simulink model "gm_sampleModel1954_3_sub"  (R2023a)
settings: Solver=VariableStepAuto  StartTime=0.0  StopTime=10.0  RelTol=1e-3
libraries: simulink x1
settings Model: Creator=user1  LastModifiedBy=user1
settings OptimizationCC: BlockReduction=off  ConditionallyExecuteInputs=off
settings DebuggingCC: InheritedTsInSrcMsg=none

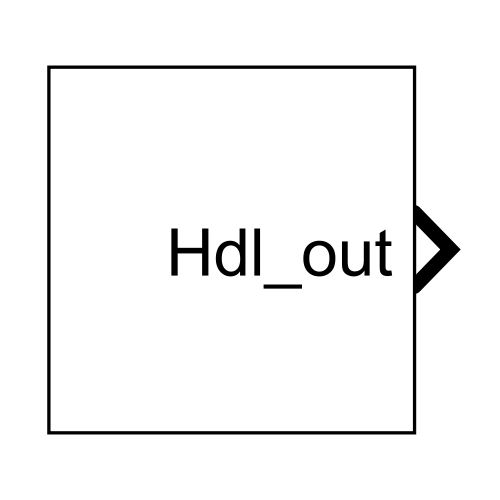
[thumbnail: Simulink's stored preview of the top-level diagram]
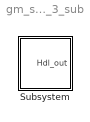
== system gm_sampleModel1954_3_sub ==
  Subsystem : Subsystem

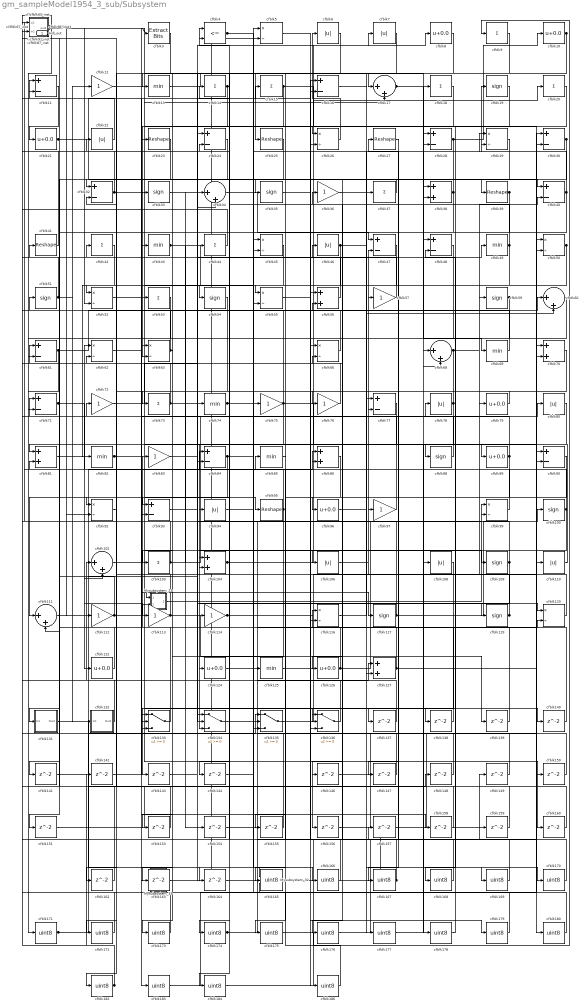
== system gm_sampleModel1954_3_sub/Subsystem ==
  Mysubsystem_23 : Subsystem
  Mysubsystem_32 : Subsystem
  Mysubsystem_33 : Subsystem
  cfblk{8,10,21,79,89,96,122,124,126} (9 alike) : Bias  Bias=0.0  SaturateOnIntegerOverflow=off
  cfblk{19,33,35,51,54,59,88,100,109,117,119} (11 alike) : Signum
  cfblk101_inst : Subsystem
  cfblk{17,34,60,68,102,111} (6 alike) : Sum  Inputs=|++  OutDataTypeStr=uint8
  cfblk{9,14..15,18,20,37,42,44,53,73,103} (11 alike) : Sum  Inputs=+  OutDataTypeStr=uint8
  cfblk{38,56,70,81,86,104,127} (7 alike) : Sum  OutDataTypeStr=uint8
  cfblk105_inst : Subsystem
  cfblk{6..7,22,46,78,80,94,106,108,110} (10 alike) : Abs  OutDataTypeStr=uint8  SaturateOnIntegerOverflow=off
  cfblk107_inst : Subsystem
  cfblk{11,16,24,28,30,32,40,47..48,61,71,77,84,90,93} (15 alike) : Sum  Inputs=+-  OutDataTypeStr=uint8
  cfblk{12,36,57,72,75..76,83,97,112..114} (11 alike) : Gain  OutDataTypeStr=uint8
  cfblk115_inst : Subsystem
  cfblk{5,26,29,45,50,52,55,62..63,66,92,99,116,120} (14 alike) : Product  Inputs=*/  OutDataTypeStr=uint8  RndMeth=Zero  SaturateOnIntegerOverflow=on
  cfblk118_inst : Subsystem
  cfblk121_inst : Subsystem
  cfblk{13,43,49,69,74,82,85,125} (8 alike) : MinMax  OutDataTypeStr=uint8
  cfblk129_inst : Subsystem
  cfblk131 : Subsystem
  cfblk132 : Subsystem
  cfblk{133..136} (4 alike) : Switch  OutDataTypeStr=uint8  SaturateOnIntegerOverflow=off  InputSameDT=off
  cfblk{137..144,146..151,153..160,162..164} (25 alike) : Delay  SampleTime=1
  cfblk{165..180,182..184,186} (20 alike) : DataTypeConversion  OutDataTypeStr=uint8  SaturateOnIntegerOverflow=off  RndMeth=Floor
  cfblk2 : Constant  Value=0  OutDataTypeStr=uint8  SampleTime=1
  cfblk{23,25,27,39,41,95} (6 alike) : Reshape
  cfblk3 : simulink/Logic and Bit Operations/Extract Bits  bitsToExtract=Upper half  numBits=8  bitIdxRange=[0 7]  outScalingMode=Preserve fixed-point scaling
      settings: LibrarySourceBlock=|
      | hdlsllib/Logic and Bit
      | Operations/Extract Bits
  cfblk31_inst : Subsystem
  cfblk4 : RelationalOperator  Operator=<=  OutDataTypeStr=boolean  InputSameDT=off
  cfblk58_inst : Subsystem
  cfblk64_inst : Subsystem
  cfblk65_inst : Subsystem
  cfblk67_inst : Subsystem
  cfblk87_inst : Subsystem
  cfblk91_inst : Subsystem
  cfblk98_inst : Subsystem
  Hdl_out : Outport  OutDataTypeStr=uint8  SampleTime=1
  wires:
  Mysubsystem_23/1(Out1) -> cfblk99/1
  Mysubsystem_32/1(Out1) -> cfblk159/1
  Mysubsystem_33/1(Out1) -> cfblk5/2
  cfblk10/1 -> cfblk25/1, cfblk55/1
  cfblk100/1 -> cfblk134/3, cfblk129_inst/1(in1)
  cfblk101_inst/1(out1) -> cfblk118_inst/1(in1)
  cfblk102/1 -> cfblk140/1
  cfblk103/1 -> cfblk78/1, cfblk58_inst/2(in2), cfblk34/1
  cfblk104/1 -> cfblk7/1, cfblk20/1
  cfblk105_inst/1(out1) -> cfblk95/1, cfblk106/1, cfblk55/2
  cfblk106/1 -> cfblk47/2
  cfblk107_inst/1(out1) -> cfblk137/1
  cfblk108/1 -> cfblk143/1
  cfblk109/1 -> cfblk124/1, cfblk105_inst/2(in2)
  cfblk11/1 -> cfblk21/1
  cfblk110/1 -> cfblk89/1
  cfblk111/1 -> cfblk86/1
  cfblk112/1 -> cfblk11/1, cfblk138/1
  cfblk113/1 -> cfblk107_inst/2(in2), cfblk139/1
  cfblk114/1 -> cfblk79/1, cfblk68/1
  cfblk115_inst/1(out1) -> cfblk91_inst/2(in2), cfblk26/1
  cfblk116/1 -> cfblk37/1
  cfblk117/1 -> cfblk121_inst/2(in2), cfblk100/1
  cfblk118_inst/1(out1) -> cfblk17/2, cfblk156/1
  cfblk119/1 -> cfblk97/1, cfblk57/1
  cfblk12/1 -> cfblk160/1
  cfblk120/1 -> cfblk72/1
  cfblk121_inst/1(out1) -> cfblk109/1
  cfblk122/1 -> cfblk71/1
  cfblk124/1 -> cfblk120/2
  cfblk125/1 -> cfblk90/1
  cfblk126/1 -> cfblk68/2, cfblk64_inst/1(in1)
  cfblk127/1 -> cfblk30/1, cfblk83/1
  cfblk129_inst/1(out1) -> cfblk180/1, cfblk104/2
  cfblk13/1 -> cfblk17/1
  cfblk131/1(Out1) -> cfblk164/1
  cfblk132/1(Out1) -> cfblk61/1
  cfblk133/1 -> cfblk107_inst/1(in1)
  cfblk134/1 -> cfblk18/1
  cfblk135/1 -> cfblk59/1
  cfblk136/1 -> cfblk102/1
  cfblk137/1 -> cfblk129_inst/2(in2)
  cfblk138/1 -> cfblk116/1
  cfblk139/1 -> cfblk81/2
  cfblk14/1 -> cfblk63/2, cfblk144/1
  cfblk140/1 -> cfblk11/2
  cfblk141/1 -> cfblk34/2
  cfblk142/1 -> cfblk77/2
  cfblk143/1 -> cfblk56/2
  cfblk144/1 -> cfblk45/2
  cfblk146/1 -> cfblk38/1
  cfblk147/1 -> cfblk62/2
  cfblk148/1 -> cfblk118_inst/2(in2)
  cfblk149/1 -> cfblk31_inst/2(in2)
  cfblk15/1 -> cfblk90/2, cfblk23/1
  cfblk150/1 -> cfblk86/2
  cfblk151/1 -> cfblk134/1
  cfblk153/1 -> cfblk32/2
  cfblk154/1 -> cfblk127/1
  cfblk155/1 -> cfblk84/1
  cfblk156/1 -> cfblk50/2
  cfblk157/1 -> cfblk30/2
  cfblk158/1 -> cfblk111/2
  cfblk159/1 -> cfblk115_inst/2(in2)
  cfblk16/1 -> cfblk60/2
  cfblk160/1 -> cfblk66/2
  cfblk162/1 -> cfblk105_inst/1(in1)
  cfblk163/1 -> cfblk99/2
  cfblk164/1 -> cfblk26/2
  cfblk165/1 -> cfblk108/1
  cfblk166/1 -> cfblk85/1
  cfblk167/1 -> cfblk67_inst/2(in2), cfblk46/1, cfblk14/1
  cfblk168/1 -> cfblk27/1
  cfblk169/1 -> cfblk56/1
  cfblk17/1 -> cfblk28/1, cfblk69/1
  cfblk170/1 -> cfblk36/1
  cfblk171/1 -> cfblk135/1, cfblk148/1
  cfblk172/1 -> cfblk65_inst/1(in1)
  cfblk173/1 -> cfblk65_inst/2(in2)
  cfblk174/1 -> cfblk110/1, cfblk157/1
  cfblk175/1 -> cfblk9/1
  cfblk176/1 -> cfblk149/1
  cfblk177/1 -> cfblk48/1
  cfblk178/1 -> cfblk48/2
  cfblk179/1 -> cfblk115_inst/1(in1)
  cfblk18/1 -> cfblk127/2
  cfblk180/1 -> cfblk5/1
  cfblk182/1 -> cfblk101_inst/1(in1), cfblk142/1
  cfblk183/1 -> cfblk70/1
  cfblk184/1 -> cfblk70/2
  cfblk186/1 -> Mysubsystem_32/2(In2)
  cfblk19/1 -> cfblk168/1
  cfblk2/1 -> cfblk98_inst/2(in2), cfblk92/2, cfblk112/1
  cfblk20/1 -> cfblk153/1
  cfblk21/1 -> cfblk38/2, cfblk15/1
  cfblk22/1 -> cfblk67_inst/1(in1)
  cfblk23/1 -> cfblk53/1
  cfblk24/1 -> cfblk162/1
  cfblk25/1 -> cfblk141/1
  cfblk26/1 -> cfblk6/1
  cfblk27/1 -> cfblk167/1
  cfblk28/1 -> cfblk133/3, cfblk10/1
  cfblk29/1 -> cfblk39/1
  cfblk3/1 -> cfblk13/1
  cfblk30/1 -> cfblk96/1, cfblk81/1
  cfblk31_inst/1(out1) -> cfblk186/1, cfblk114/1
  cfblk32/1 -> cfblk98_inst/1(in1), cfblk54/1, cfblk172/1, cfblk75/1
  cfblk33/1 -> cfblk119/1
  cfblk34/1 -> cfblk77/1
  cfblk35/1 -> cfblk47/1
  cfblk36/1 -> cfblk169/1
  cfblk37/1 -> cfblk33/1
  cfblk38/1 -> cfblk35/1, cfblk134/2
  cfblk39/1 -> cfblk135/2, cfblk151/1
  cfblk4/1 -> cfblk40/1, cfblk166/1
  cfblk40/1 -> cfblk19/1, cfblk104/1
  cfblk41/1 -> cfblk31_inst/1(in1)
  cfblk42/1 -> cfblk82/1
  cfblk43/1 -> cfblk135/3, cfblk154/1, cfblk125/1
  cfblk44/1 -> cfblk87_inst/2(in2)
  cfblk45/1 -> cfblk94/1
  cfblk46/1 -> cfblk29/2, cfblk150/1, Mysubsystem_23/1(In1)
  cfblk47/1 -> cfblk93/1
  cfblk48/1 -> cfblk176/1
  cfblk49/1 -> cfblk22/1, cfblk52/1
  cfblk5/1 -> cfblk179/1
  cfblk50/1 -> cfblk175/1, cfblk92/1, cfblk63/1
  cfblk51/1 -> cfblk64_inst/2(in2), cfblk12/1, cfblk132/1(In1)
  cfblk52/1 -> cfblk183/1
  cfblk53/1 -> cfblk61/2
  cfblk54/1 -> cfblk103/1
  cfblk55/1 -> cfblk16/2
  cfblk56/1 -> cfblk41/1
  cfblk57/1 -> cfblk24/2
  cfblk58_inst/1(out1) -> Mysubsystem_33/1(In1)
  cfblk59/1 -> cfblk136/2, cfblk147/1, cfblk146/1
  cfblk6/1 -> cfblk32/1
  cfblk60/1 -> cfblk133/2
  cfblk61/1 -> cfblk71/2, cfblk50/1
  cfblk62/1 -> cfblk117/1
  cfblk63/1 -> cfblk58_inst/1(in1), cfblk173/1
  cfblk64_inst/1(out1) -> cfblk121_inst/1(in1), Mysubsystem_23/2(In2)
  cfblk65_inst/1(out1) -> cfblk171/1
  cfblk66/1 -> cfblk51/1
  cfblk67_inst/1(out1) -> cfblk74/1
  cfblk68/1 -> cfblk88/1, cfblk40/2, cfblk184/1
  cfblk69/1 -> cfblk4/1
  cfblk7/1 -> cfblk43/1
  cfblk70/1 -> cfblk182/1
  cfblk71/1 -> cfblk102/2, cfblk113/1
  cfblk72/1 -> cfblk44/1
  cfblk73/1 -> cfblk101_inst/2(in2), cfblk49/1
  cfblk74/1 -> cfblk136/1, cfblk120/1
  cfblk75/1 -> cfblk4/2, cfblk178/1, cfblk131/1(In1)
  cfblk76/1 -> cfblk87_inst/1(in1)
  cfblk77/1 -> cfblk84/2
  cfblk78/1 -> cfblk126/1, cfblk76/1
  cfblk79/1 -> cfblk73/1
  cfblk8/1 -> cfblk133/1
  cfblk80/1 -> cfblk93/2
  cfblk81/1 -> cfblk122/1
  cfblk82/1 -> cfblk16/1, cfblk158/1, Mysubsystem_32/1(In1)
  cfblk83/1 -> cfblk80/1
  cfblk84/1 -> cfblk111/1, cfblk29/1
  cfblk85/1 -> cfblk165/1
  cfblk86/1 -> cfblk116/2
  cfblk87_inst/1(out1) -> cfblk177/1
  cfblk88/1 -> cfblk66/1
  cfblk89/1 -> cfblk91_inst/1(in1), cfblk136/3
  cfblk9/1 -> cfblk174/1
  cfblk90/1 -> cfblk155/1
  cfblk91_inst/1(out1) -> cfblk28/2, cfblk52/2
  cfblk92/1 -> cfblk42/1
  cfblk93/1 -> cfblk8/1
  cfblk94/1 -> cfblk60/1
  cfblk95/1 -> cfblk24/1, cfblk163/1
  cfblk96/1 -> cfblk170/1
  cfblk97/1 -> cfblk45/1
  cfblk98_inst/1(out1) -> cfblk3/1, Hdl_out/1
  cfblk99/1 -> cfblk62/1

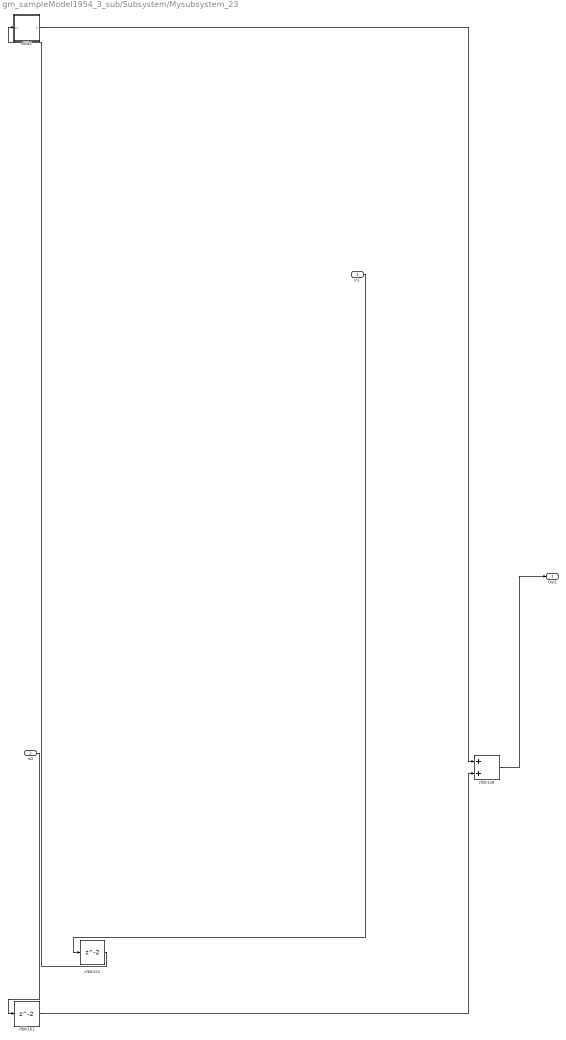
== system gm_sampleModel1954_3_sub/Subsystem/Mysubsystem_23 ==
  In1 : Inport  OutDataTypeStr=uint8  PortDimensions=1  SampleTime=1
  In2 : Inport  Port=2  OutDataTypeStr=uint8  PortDimensions=1  SampleTime=1
  cfblk1 : Subsystem  mask(Detect Fall Nonpositive){vinit=double(0), InputProcessing=Elements as channels (sample based), OutDataTypeStr=boolean}
      mask prompts: vinit "Simulink:masks:InitialCondition_MP"; InputProcessing "Simulink:masks:InputProcessing_MP"; OutDataTypeStr "Simulink:masks:OutputDataType_MP"
      mask help: Simulink:masks:DetectFallNonpositive_MD
      mask init:
      | InputProcessing = 'Elements as channels (sample based)';
      | OutDataTypeStr = 'boolean';
      | vinit = double(0);
      mask TypeOptions InputProcessing: Simulink:masks:ColumnsAsChannelsFrameBased | Simulink:masks:ElementsAsChannelsSampleBased
      mask TypeOptions OutDataTypeStr: Simulink:masks:uint8 | Simulink:masks:boolean
      mask Display: fprintf('U <= 0\n&  NOT\nU/z <= 0')
  cfblk128 : Sum
  cfblk152 : Delay  SampleTime=1
  cfblk161 : Delay  SampleTime=1
  Out1 : Outport  SampleTime=1
  wires:
  In1/1 -> cfblk152/1
  In2/1 -> cfblk161/1
  cfblk1/1(Y) -> cfblk128/1
  cfblk128/1 -> Out1/1
  cfblk152/1 -> cfblk1/1(U)
  cfblk161/1 -> cfblk128/2

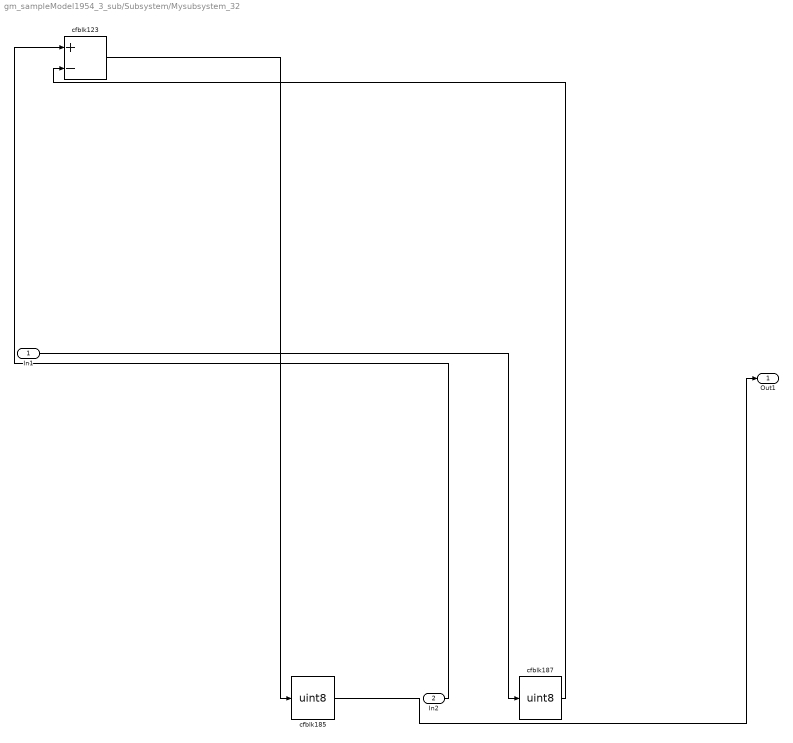
== system gm_sampleModel1954_3_sub/Subsystem/Mysubsystem_32 ==
  In1 : Inport  OutDataTypeStr=uint8  PortDimensions=1  SampleTime=1
  In2 : Inport  Port=2  OutDataTypeStr=uint8  PortDimensions=1  SampleTime=1
  cfblk123 : Sum  Inputs=+-
  cfblk185 : DataTypeConversion  OutDataTypeStr=uint8  SaturateOnIntegerOverflow=off  RndMeth=Floor
  cfblk187 : DataTypeConversion  OutDataTypeStr=uint8  SaturateOnIntegerOverflow=off  RndMeth=Floor
  Out1 : Outport  SampleTime=1
  wires:
  In1/1 -> cfblk187/1
  In2/1 -> cfblk123/1
  cfblk123/1 -> cfblk185/1
  cfblk185/1 -> Out1/1
  cfblk187/1 -> cfblk123/2

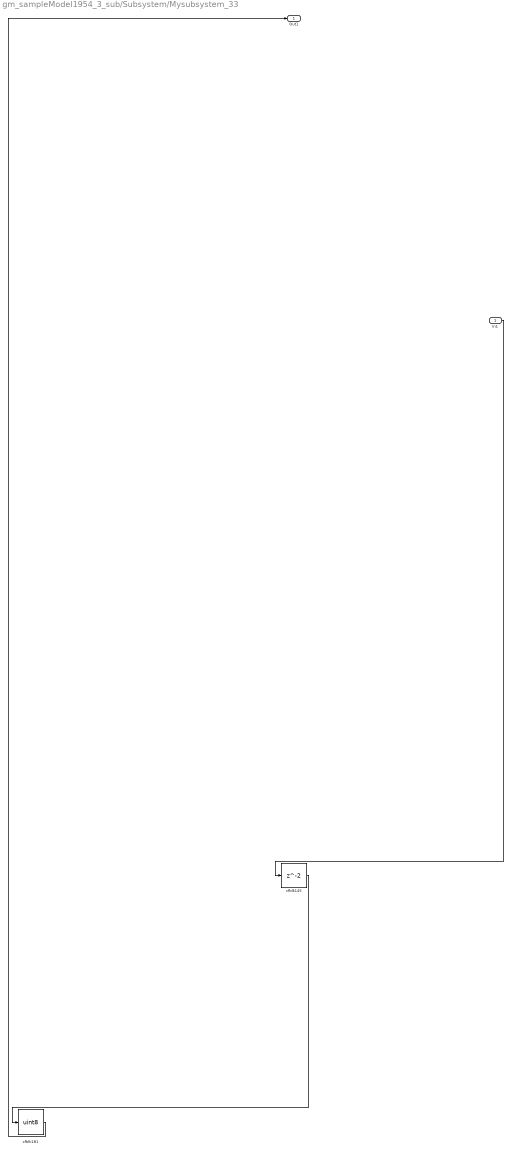
== system gm_sampleModel1954_3_sub/Subsystem/Mysubsystem_33 ==
  In1 : Inport  OutDataTypeStr=uint8  PortDimensions=1  SampleTime=1
  cfblk145 : Delay  SampleTime=1
  cfblk181 : DataTypeConversion  OutDataTypeStr=uint8  SaturateOnIntegerOverflow=off  RndMeth=Floor
  Out1 : Outport  SampleTime=1
  wires:
  In1/1 -> cfblk145/1
  cfblk145/1 -> cfblk181/1
  cfblk181/1 -> Out1/1

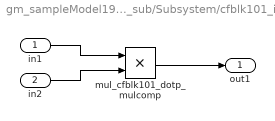
== system gm_sampleModel1954_3_sub/Subsystem/cfblk101_inst ==
  in1 : Inport  OutDataTypeStr=uint8  SampleTime=1
  in2 : Inport  Port=2  OutDataTypeStr=uint8  SampleTime=1
  mul_cfblk101_dotp_mulcomp : Product  Inputs=**  OutDataTypeStr=uint8  SampleTime=1
  out1 : Outport  OutDataTypeStr=uint8  SampleTime=1
  wires:
  in1/1 -> mul_cfblk101_dotp_mulcomp/1
  in2/1 -> mul_cfblk101_dotp_mulcomp/2
  mul_cfblk101_dotp_mulcomp/1 -> out1/1

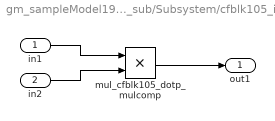
== system gm_sampleModel1954_3_sub/Subsystem/cfblk105_inst ==
  in1 : Inport  OutDataTypeStr=uint8  SampleTime=1
  in2 : Inport  Port=2  OutDataTypeStr=uint8  SampleTime=1
  mul_cfblk105_dotp_mulcomp : Product  Inputs=**  OutDataTypeStr=uint8  SampleTime=1
  out1 : Outport  OutDataTypeStr=uint8  SampleTime=1
  wires:
  in1/1 -> mul_cfblk105_dotp_mulcomp/1
  in2/1 -> mul_cfblk105_dotp_mulcomp/2
  mul_cfblk105_dotp_mulcomp/1 -> out1/1

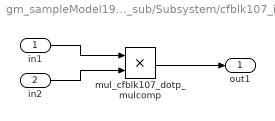
== system gm_sampleModel1954_3_sub/Subsystem/cfblk107_inst ==
  in1 : Inport  OutDataTypeStr=uint8  SampleTime=1
  in2 : Inport  Port=2  OutDataTypeStr=uint8  SampleTime=1
  mul_cfblk107_dotp_mulcomp : Product  Inputs=**  OutDataTypeStr=uint8  SampleTime=1
  out1 : Outport  OutDataTypeStr=uint8  SampleTime=1
  wires:
  in1/1 -> mul_cfblk107_dotp_mulcomp/1
  in2/1 -> mul_cfblk107_dotp_mulcomp/2
  mul_cfblk107_dotp_mulcomp/1 -> out1/1

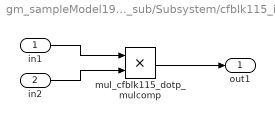
== system gm_sampleModel1954_3_sub/Subsystem/cfblk115_inst ==
  in1 : Inport  OutDataTypeStr=uint8  SampleTime=1
  in2 : Inport  Port=2  OutDataTypeStr=uint8  SampleTime=1
  mul_cfblk115_dotp_mulcomp : Product  Inputs=**  OutDataTypeStr=uint8  SampleTime=1
  out1 : Outport  OutDataTypeStr=uint8  SampleTime=1
  wires:
  in1/1 -> mul_cfblk115_dotp_mulcomp/1
  in2/1 -> mul_cfblk115_dotp_mulcomp/2
  mul_cfblk115_dotp_mulcomp/1 -> out1/1

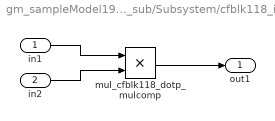
== system gm_sampleModel1954_3_sub/Subsystem/cfblk118_inst ==
  in1 : Inport  OutDataTypeStr=uint8  SampleTime=1
  in2 : Inport  Port=2  OutDataTypeStr=uint8  SampleTime=1
  mul_cfblk118_dotp_mulcomp : Product  Inputs=**  OutDataTypeStr=uint8  SampleTime=1
  out1 : Outport  OutDataTypeStr=uint8  SampleTime=1
  wires:
  in1/1 -> mul_cfblk118_dotp_mulcomp/1
  in2/1 -> mul_cfblk118_dotp_mulcomp/2
  mul_cfblk118_dotp_mulcomp/1 -> out1/1

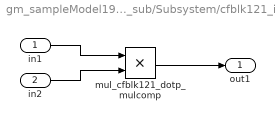
== system gm_sampleModel1954_3_sub/Subsystem/cfblk121_inst ==
  in1 : Inport  OutDataTypeStr=uint8  SampleTime=1
  in2 : Inport  Port=2  OutDataTypeStr=uint8  SampleTime=1
  mul_cfblk121_dotp_mulcomp : Product  Inputs=**  OutDataTypeStr=uint8  SampleTime=1
  out1 : Outport  OutDataTypeStr=uint8  SampleTime=1
  wires:
  in1/1 -> mul_cfblk121_dotp_mulcomp/1
  in2/1 -> mul_cfblk121_dotp_mulcomp/2
  mul_cfblk121_dotp_mulcomp/1 -> out1/1

== system gm_sampleModel1954_3_sub/Subsystem/cfblk129_inst ==
  in1 : Inport  OutDataTypeStr=uint8  SampleTime=1
  in2 : Inport  Port=2  OutDataTypeStr=uint8  SampleTime=1
  mul_cfblk129_dotp_mulcomp : Product  Inputs=**  OutDataTypeStr=uint8  SampleTime=1
  out1 : Outport  OutDataTypeStr=uint8  SampleTime=1
  wires:
  in1/1 -> mul_cfblk129_dotp_mulcomp/1
  in2/1 -> mul_cfblk129_dotp_mulcomp/2
  mul_cfblk129_dotp_mulcomp/1 -> out1/1

== system gm_sampleModel1954_3_sub/Subsystem/cfblk131 ==
  In1 : Inport  OutDataTypeStr=uint8  PortDimensions=1  SampleTime=1
  Out1 : Outport  SampleTime=1
  wires:
  In1/1 -> Out1/1

== system gm_sampleModel1954_3_sub/Subsystem/cfblk132 ==
  In1 : Inport  OutDataTypeStr=uint8  PortDimensions=1  SampleTime=1
  Out1 : Outport  SampleTime=1
  wires:
  In1/1 -> Out1/1

== system gm_sampleModel1954_3_sub/Subsystem/cfblk31_inst ==
  in1 : Inport  OutDataTypeStr=uint8  SampleTime=1
  in2 : Inport  Port=2  OutDataTypeStr=uint8  SampleTime=1
  mul_cfblk31_dotp_mulcomp : Product  Inputs=**  OutDataTypeStr=uint8  SampleTime=1
  out1 : Outport  OutDataTypeStr=uint8  SampleTime=1
  wires:
  in1/1 -> mul_cfblk31_dotp_mulcomp/1
  in2/1 -> mul_cfblk31_dotp_mulcomp/2
  mul_cfblk31_dotp_mulcomp/1 -> out1/1

== system gm_sampleModel1954_3_sub/Subsystem/cfblk58_inst ==
  in1 : Inport  OutDataTypeStr=uint8  SampleTime=1
  in2 : Inport  Port=2  OutDataTypeStr=uint8  SampleTime=1
  mul_cfblk58_dotp_mulcomp : Product  Inputs=**  OutDataTypeStr=uint8  SampleTime=1
  out1 : Outport  OutDataTypeStr=uint8  SampleTime=1
  wires:
  in1/1 -> mul_cfblk58_dotp_mulcomp/1
  in2/1 -> mul_cfblk58_dotp_mulcomp/2
  mul_cfblk58_dotp_mulcomp/1 -> out1/1

== system gm_sampleModel1954_3_sub/Subsystem/cfblk64_inst ==
  in1 : Inport  OutDataTypeStr=uint8  SampleTime=1
  in2 : Inport  Port=2  OutDataTypeStr=uint8  SampleTime=1
  mul_cfblk64_dotp_mulcomp : Product  Inputs=**  OutDataTypeStr=uint8  SampleTime=1
  out1 : Outport  OutDataTypeStr=uint8  SampleTime=1
  wires:
  in1/1 -> mul_cfblk64_dotp_mulcomp/1
  in2/1 -> mul_cfblk64_dotp_mulcomp/2
  mul_cfblk64_dotp_mulcomp/1 -> out1/1

== system gm_sampleModel1954_3_sub/Subsystem/cfblk65_inst ==
  in1 : Inport  OutDataTypeStr=uint8  SampleTime=1
  in2 : Inport  Port=2  OutDataTypeStr=uint8  SampleTime=1
  mul_cfblk65_dotp_mulcomp : Product  Inputs=**  OutDataTypeStr=uint8  SampleTime=1
  out1 : Outport  OutDataTypeStr=uint8  SampleTime=1
  wires:
  in1/1 -> mul_cfblk65_dotp_mulcomp/1
  in2/1 -> mul_cfblk65_dotp_mulcomp/2
  mul_cfblk65_dotp_mulcomp/1 -> out1/1

== system gm_sampleModel1954_3_sub/Subsystem/cfblk67_inst ==
  in1 : Inport  OutDataTypeStr=uint8  SampleTime=1
  in2 : Inport  Port=2  OutDataTypeStr=uint8  SampleTime=1
  mul_cfblk67_dotp_mulcomp : Product  Inputs=**  OutDataTypeStr=uint8  SampleTime=1
  out1 : Outport  OutDataTypeStr=uint8  SampleTime=1
  wires:
  in1/1 -> mul_cfblk67_dotp_mulcomp/1
  in2/1 -> mul_cfblk67_dotp_mulcomp/2
  mul_cfblk67_dotp_mulcomp/1 -> out1/1

== system gm_sampleModel1954_3_sub/Subsystem/cfblk87_inst ==
  in1 : Inport  OutDataTypeStr=uint8  SampleTime=1
  in2 : Inport  Port=2  OutDataTypeStr=uint8  SampleTime=1
  mul_cfblk87_dotp_mulcomp : Product  Inputs=**  OutDataTypeStr=uint8  SampleTime=1
  out1 : Outport  OutDataTypeStr=uint8  SampleTime=1
  wires:
  in1/1 -> mul_cfblk87_dotp_mulcomp/1
  in2/1 -> mul_cfblk87_dotp_mulcomp/2
  mul_cfblk87_dotp_mulcomp/1 -> out1/1

== system gm_sampleModel1954_3_sub/Subsystem/cfblk91_inst ==
  in1 : Inport  OutDataTypeStr=uint8  SampleTime=1
  in2 : Inport  Port=2  OutDataTypeStr=uint8  SampleTime=1
  mul_cfblk91_dotp_mulcomp : Product  Inputs=**  OutDataTypeStr=uint8  SampleTime=1
  out1 : Outport  OutDataTypeStr=uint8  SampleTime=1
  wires:
  in1/1 -> mul_cfblk91_dotp_mulcomp/1
  in2/1 -> mul_cfblk91_dotp_mulcomp/2
  mul_cfblk91_dotp_mulcomp/1 -> out1/1

== system gm_sampleModel1954_3_sub/Subsystem/cfblk98_inst ==
  in1 : Inport  OutDataTypeStr=uint8  SampleTime=1
  in2 : Inport  Port=2  OutDataTypeStr=uint8  SampleTime=1
  mul_cfblk98_dotp_mulcomp : Product  Inputs=**  OutDataTypeStr=uint8  SampleTime=1
  out1 : Outport  OutDataTypeStr=uint8  SampleTime=1
  wires:
  in1/1 -> mul_cfblk98_dotp_mulcomp/1
  in2/1 -> mul_cfblk98_dotp_mulcomp/2
  mul_cfblk98_dotp_mulcomp/1 -> out1/1

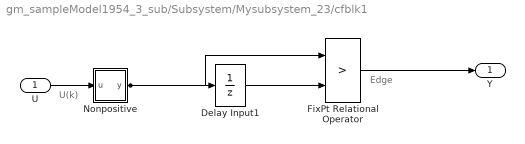
== system gm_sampleModel1954_3_sub/Subsystem/Mysubsystem_23/cfblk1 ==
  note: U(k)
  note: Edge
  U : Inport  OutDataTypeStr=uint8  SampleTime=1
  Delay Input1 : UnitDelay  Description=Store in Global RAM  DisableCoverage=on  InitialCondition=vinit  SampleTime=-1  HasFrameUpgradeWarning=on
  FixPt Relational Operator : RelationalOperator  Operator=>  OutDataTypeStr=boolean  ZeroCross=off  InputSameDT=off
  Nonpositive : Subsystem  mask(Compare To Zero){relop=<=, OutDataTypeStr=boolean, ZeroCross=off}
      mask prompts: relop "Simulink:masks:Operator_MP"; OutDataTypeStr "Simulink:masks:OutputDataType_MP"; ZeroCross "Simulink:masks:EnableZerocrossingDetection_MP"
      mask help: Simulink:masks:CompareToZero_MD
      mask init:
      | OutDataTypeStr = 'boolean';
      | ZeroCross = 'off';
      | blkName = 'sampleModel1954_3_sub/Subsystem/Mysubsystem_23/cfblk1/Nonpositive';
      | relop = '<=';
      | setValue = 'boolean';
      mask TypeOptions relop: == | ~= | < | <= | >= | >
      mask TypeOptions OutDataTypeStr: Simulink:masks:uint8 | Simulink:masks:boolean
      mask Callback ZeroCross: sl('zeroCrossEnable', gcbh);
      mask Display: disp([relop,' 0'])
  Y : Outport  SampleTime=1
  wires:
  U/1 -> Nonpositive/1(u)
  Delay Input1/1 -> FixPt Relational Operator/2
  FixPt Relational Operator/1 -> Y/1
  Nonpositive/1(y) -> FixPt Relational Operator/1, Delay Input1/1

== system gm_sampleModel1954_3_sub/Subsystem/Mysubsystem_23/cfblk1/Nonpositive ==
  u : Inport  OutDataTypeStr=uint8  SampleTime=1
  Compare : RelationalOperator  Operator=<=  OutDataTypeStr=boolean  ZeroCross=off
  Constant : Constant  DisableCoverage=on  Value=0  OutDataTypeStr=Inherit: Inherit via back propagation  SampleTime=-1  PreserveConstantTs=on
  y : Outport  SampleTime=1
  wires:
  u/1 -> Compare/1
  Compare/1 -> y/1
  Constant/1 -> Compare/2
